simulink model "Simulink_11_Nov"  (R2020a)
settings: Solver=VariableStepAuto  StartTime=0.0  StopTime=50  RelTol=1e-3
libraries: cstblocks x10
settings Model: Creator=geral  LastModifiedBy=geral

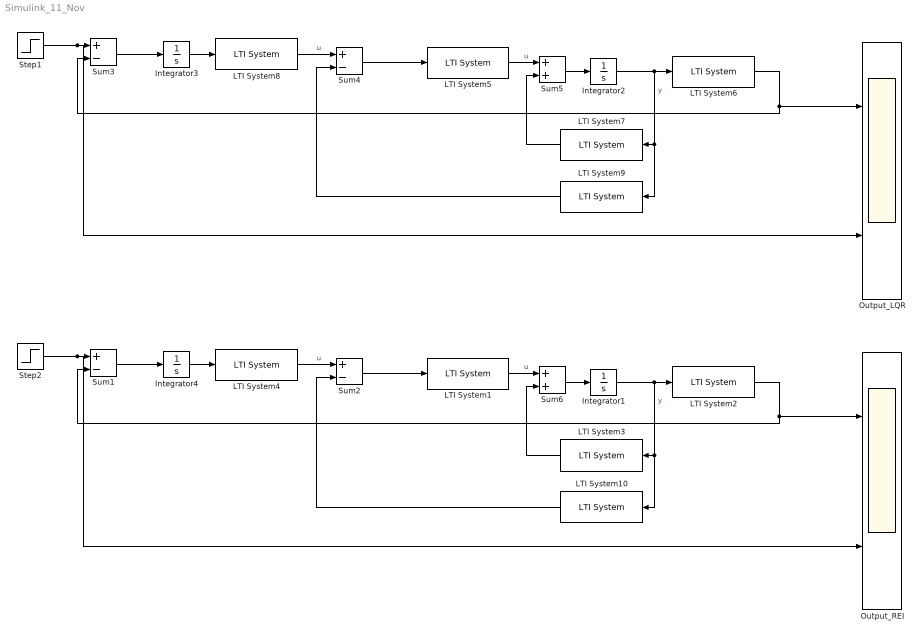
== system Simulink_11_Nov ==
  Integrator{1..4} (4 alike) : Integrator
  LTI System1 : cstblocks/LTI System  sys=Heli_ss.B  IC=[]
  LTI System10 : cstblocks/LTI System  sys=K_REI  IC=[]
  LTI System2 : cstblocks/LTI System  sys=[1 0 0 0]  IC=[]
  LTI System3 : cstblocks/LTI System  sys=Heli_ss.A  IC=[]
  LTI System4 : cstblocks/LTI System  sys=Ki_REI  IC=[]
  LTI System5 : cstblocks/LTI System  sys=Heli_ss.B  IC=[]
  LTI System6 : cstblocks/LTI System  sys=[1 0 0 0]  IC=[]
  LTI System7 : cstblocks/LTI System  sys=Heli_ss.A  IC=[]
  LTI System8 : cstblocks/LTI System  sys=Ki_LQR  IC=[]
  LTI System9 : cstblocks/LTI System  sys=K_LQR  IC=[]
  Output_LQR : Scope  NumInputPorts=2
  Output_REI : Scope  NumInputPorts=2
  Step1 : Step  Time=0.1  After=0.583  SampleTime=0
  Step2 : Step  Time=0.1  After=0.583  SampleTime=0
  Sum{1..4} (4 alike) : Sum  Inputs=+-
  Sum5 : Sum
  Sum6 : Sum
  wires:
  LTI System5/1 -> Sum5/1  "u"
  Integrator3/1 -> LTI System8/1
  LTI System7/1 -> Sum5/2
  LTI System8/1 -> Sum4/1  "u"
  Step1/1 -> Output_LQR/2, Sum3/1
  LTI System6/1 -> Sum3/2, Output_LQR/1
  Sum3/1 -> Integrator3/1
  Integrator2/1 -> LTI System6/1, LTI System9/1, LTI System7/1  "y"
  Sum5/1 -> Integrator2/1
  LTI System9/1 -> Sum4/2
  Sum4/1 -> LTI System5/1
  Sum6/1 -> Integrator1/1
  Integrator1/1 -> LTI System2/1, LTI System10/1, LTI System3/1  "y"
  LTI System4/1 -> Sum2/1  "u"
  LTI System2/1 -> Sum1/2, Output_REI/1
  Step2/1 -> Output_REI/2, Sum1/1
  Sum1/1 -> Integrator4/1
  LTI System1/1 -> Sum6/1  "u"
  LTI System10/1 -> Sum2/2
  Sum2/1 -> LTI System1/1
  Integrator4/1 -> LTI System4/1
  LTI System3/1 -> Sum6/2
